simulink model "ResonantConverter_GaN"  (R2016a)
settings: Solver=VariableStepAuto  StartTime=0.0  StopTime=0.1  FixedStep=1e-6  RelTol=1e-3
libraries: powerlib x142, dspstat3 x22, powerlib_meascontrol x13
(part 2 of 2)

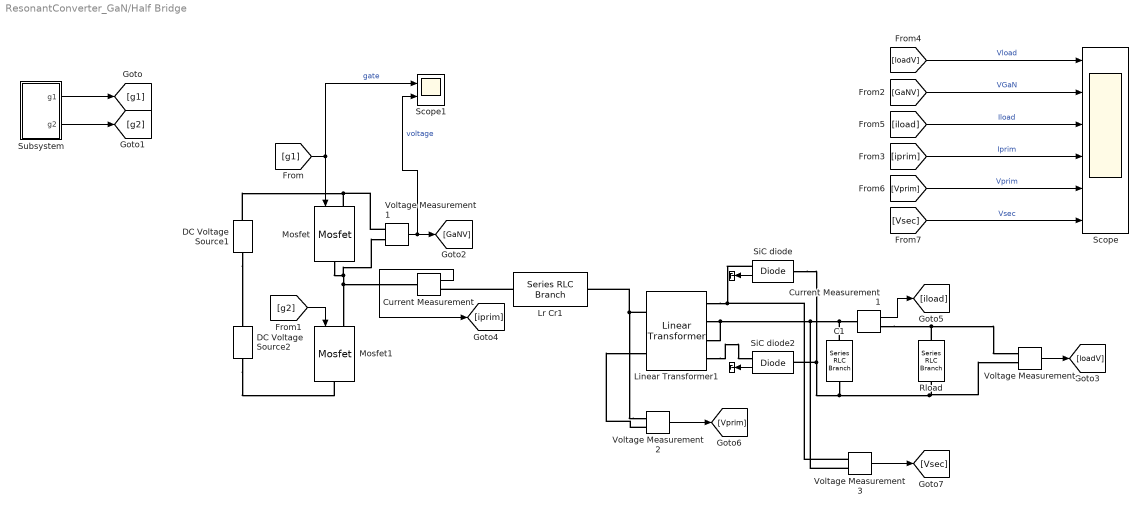
== system ResonantConverter_GaN/Half Bridge ==
  "  " : Terminator
  "   " : Terminator
  C1 : powerlib/Elements/Series RLC Branch  LConnTagsString=__new0  RConnTagsString=__new0  BranchType=C  Resistance=1  Inductance=1e-3  SetiL0=off  InitialCurrent=0  Capacitance=1e-6  Setx0=off  InitialVoltage=0  Measurements=None
  Current Measurement : powerlib/Measurements/Current Measurement  PhasorSimulation=off  OutputType=Complex  PSBequivalent=0
  Current Measurement1 : powerlib/Measurements/Current Measurement  PhasorSimulation=off  OutputType=Complex  PSBequivalent=0
  DC Voltage Source1 : powerlib/Electrical Sources/DC Voltage Source  Amplitude=190  Measurements=None
  DC Voltage Source2 : powerlib/Electrical Sources/DC Voltage Source  Amplitude=190  Measurements=None
  Linear Transformer1 : powerlib/Elements/Linear Transformer  UNITS=SI  NominalPower=[ 400 250e3 ]  winding1=[380 0.1805 4.5964e-06]  winding2=[380 0.1805 4.5964e-06]  ThreeWindings=on  winding3=[380 0.1805 4.5964e-06]  RmLm=[4e6 118e-06]  Measurements=None  DataType=on
  Lr Cr1 : powerlib/Elements/Series RLC Branch  LConnTagsString=__new0  RConnTagsString=__new0  BranchType=LC  Resistance=1  Inductance=100e-6  SetiL0=off  InitialCurrent=0  Capacitance=4.053e-10  Setx0=off  InitialVoltage=0  Measurements=None
  Mosfet : powerlib/Power Electronics/Mosfet  Ron=130e-3  Lon=0  Rd=0.25  Vfd=2.2  IC=0  Rs=1e5  Cs=inf  Measurements=off
  Mosfet1 : powerlib/Power Electronics/Mosfet  Ron=130e-3  Lon=0  Rd=0.25  Vfd=2.2  IC=0  Rs=1e5  Cs=inf  Measurements=off
  Rload : powerlib/Elements/Series RLC Branch  LConnTagsString=__new0  RConnTagsString=__new0  BranchType=R  Resistance=6  Inductance=1e-3  SetiL0=off  InitialCurrent=0  Capacitance=1e-6  Setx0=off  InitialVoltage=0  Measurements=None
  Scope : Scope  NumInputPorts=6
  Scope1 : Scope  NumInputPorts=2
  SiC diode : powerlib/Power Electronics/Diode  Ron=0.001  Lon=0  Vf=0.8  IC=0  UseSnubber=off  Rs=500  Cs=250e-9  Measurements=on
  SiC diode2 : powerlib/Power Electronics/Diode  Ron=0.001  Lon=0  Vf=0.8  IC=0  UseSnubber=off  Rs=500  Cs=250e-9  Measurements=on
  Subsystem : Subsystem
  Voltage Measurement{,1..3} (4 alike) : powerlib/Measurements/Voltage Measurement  PhasorSimulation=off  OutputType=Complex  PSBequivalent=0
  wires:
  Voltage Measurement/1 -> [loadV]
  [loadV] -> Scope/1  "Vload"
  [g2] -> Mosfet1/1
  [iprim] -> Scope/4  "Iprim"
  [g1] -> Mosfet/1, Scope1/1  "gate"
  Current Measurement1/1 -> [iload]
  [GaNV] -> Scope/2  "VGaN"
  Current Measurement/1 -> [iprim]
  SiC diode/1 -> "  "/1
  SiC diode2/1 -> "   "/1
  [iload] -> Scope/3  "Iload"
  Voltage Measurement1/1 -> [GaNV], Scope1/2  "voltage"
  Subsystem/1("g1 ") -> [g1]
  Subsystem/2(g2) -> [g2]
  Voltage Measurement2/1 -> [Vprim]
  [Vprim] -> Scope/5  "Vprim"
  Voltage Measurement3/1 -> [Vsec]
  [Vsec] -> Scope/6  "Vsec"
  connections:
  Linear Transformer1/RConn4 -- SiC diode2/RConn1
  Voltage Measurement2/LConn1 -- Linear Transformer1/LConn1 -- Lr Cr1/RConn1
  SiC diode/RConn1 -- Linear Transformer1/RConn1 -- Voltage Measurement3/LConn1
  SiC diode/LConn1 -- SiC diode2/LConn1 -- C1/RConn1 -- Voltage Measurement/LConn2 -- Rload/RConn1
  Voltage Measurement1/LConn1 -- DC Voltage Source1/RConn1 -- Mosfet/LConn1
  Rload/LConn1 -- Current Measurement1/RConn1 -- Voltage Measurement/LConn1
  Mosfet/RConn1 -- Mosfet1/LConn1 -- Current Measurement/LConn1 -- Voltage Measurement1/LConn2
  Linear Transformer1/RConn3 -- Linear Transformer1/RConn2 -- Voltage Measurement3/LConn2 -- C1/LConn1 -- Current Measurement1/LConn1
  Voltage Measurement2/LConn2 -- Linear Transformer1/LConn2
  Lr Cr1/LConn1 -- Current Measurement/RConn1
  DC Voltage Source1/LConn1 -- DC Voltage Source2/RConn1
  DC Voltage Source2/LConn1 -- Mosfet1/RConn1

== system ResonantConverter_GaN/230 khz Switch1/Subsystem ==
  Constant : Constant
  Constant1 : Constant  Value=0
  Constant2 : Constant  Value=0
  Constant3 : Constant
  Sawtooth Generator : powerlib_meascontrol/Pulse & Signal Generators/Sawtooth Generator  Freq=230e3  Phase=180  Ts=0
  Scope : Scope
  Switch : Switch  Criteria=u2 > Threshold
  Switch1 : Switch
  "g1 " : Outport
  g2 : Outport  Port=2
  wires:
  Constant/1 -> Switch/1
  Constant3/1 -> Switch1/3
  Constant1/1 -> Switch/3
  Constant2/1 -> Switch1/1
  Switch/1 -> "g1 "/1, Scope/1
  Sawtooth Generator/1 -> Switch/2, Switch1/2
  Switch1/1 -> g2/1

== system ResonantConverter_GaN/235 khz Switch3/Subsystem ==
  Constant : Constant
  Constant1 : Constant  Value=0
  Constant2 : Constant  Value=0
  Constant3 : Constant
  Sawtooth Generator : powerlib_meascontrol/Pulse & Signal Generators/Sawtooth Generator  Freq=235e3  Phase=180  Ts=0
  Scope : Scope
  Switch : Switch  Criteria=u2 > Threshold
  Switch1 : Switch
  "g1 " : Outport
  g2 : Outport  Port=2
  wires:
  Constant/1 -> Switch/1
  Constant3/1 -> Switch1/3
  Constant1/1 -> Switch/3
  Constant2/1 -> Switch1/1
  Switch/1 -> "g1 "/1, Scope/1
  Sawtooth Generator/1 -> Switch/2, Switch1/2
  Switch1/1 -> g2/1

== system ResonantConverter_GaN/238 khz Switch2/Subsystem ==
  Constant : Constant
  Constant1 : Constant  Value=0
  Constant2 : Constant  Value=0
  Constant3 : Constant
  Sawtooth Generator : powerlib_meascontrol/Pulse & Signal Generators/Sawtooth Generator  Freq=238e3  Phase=180  Ts=0
  Scope : Scope
  Switch : Switch  Criteria=u2 > Threshold
  Switch1 : Switch
  "g1 " : Outport
  g2 : Outport  Port=2
  wires:
  Switch1/1 -> g2/1
  Sawtooth Generator/1 -> Switch1/2, Switch/2
  Switch/1 -> Scope/1, "g1 "/1
  Constant2/1 -> Switch1/1
  Constant1/1 -> Switch/3
  Constant3/1 -> Switch1/3
  Constant/1 -> Switch/1

== system ResonantConverter_GaN/240 khz Switch2/Subsystem ==
  Constant : Constant
  Constant1 : Constant  Value=0
  Constant2 : Constant  Value=0
  Constant3 : Constant
  Sawtooth Generator : powerlib_meascontrol/Pulse & Signal Generators/Sawtooth Generator  Freq=240e3  Phase=180  Ts=0
  Scope : Scope
  Switch : Switch  Criteria=u2 > Threshold
  Switch1 : Switch
  "g1 " : Outport
  g2 : Outport  Port=2
  wires:
  Switch1/1 -> g2/1
  Sawtooth Generator/1 -> Switch1/2, Switch/2
  Switch/1 -> Scope/1, "g1 "/1
  Constant2/1 -> Switch1/1
  Constant1/1 -> Switch/3
  Constant3/1 -> Switch1/3
  Constant/1 -> Switch/1

== system ResonantConverter_GaN/241 khz Switch1/Subsystem ==
  Constant : Constant
  Constant1 : Constant  Value=0
  Constant2 : Constant  Value=0
  Constant3 : Constant
  Sawtooth Generator : powerlib_meascontrol/Pulse & Signal Generators/Sawtooth Generator  Freq=241e3  Phase=180  Ts=0
  Scope : Scope
  Switch : Switch  Criteria=u2 > Threshold
  Switch1 : Switch
  "g1 " : Outport
  g2 : Outport  Port=2
  wires:
  Switch1/1 -> g2/1
  Sawtooth Generator/1 -> Switch1/2, Switch/2
  Switch/1 -> Scope/1, "g1 "/1
  Constant2/1 -> Switch1/1
  Constant1/1 -> Switch/3
  Constant3/1 -> Switch1/3
  Constant/1 -> Switch/1

== system ResonantConverter_GaN/244 khz Switch1/Subsystem ==
  Constant : Constant
  Constant1 : Constant  Value=0
  Constant2 : Constant  Value=0
  Constant3 : Constant
  Sawtooth Generator : powerlib_meascontrol/Pulse & Signal Generators/Sawtooth Generator  Freq=244e3  Phase=180  Ts=0
  Scope : Scope
  Switch : Switch  Criteria=u2 > Threshold
  Switch1 : Switch
  "g1 " : Outport
  g2 : Outport  Port=2
  wires:
  Constant/1 -> Switch/1
  Constant3/1 -> Switch1/3
  Constant1/1 -> Switch/3
  Constant2/1 -> Switch1/1
  Switch/1 -> "g1 "/1, Scope/1
  Sawtooth Generator/1 -> Switch/2, Switch1/2
  Switch1/1 -> g2/1

== system ResonantConverter_GaN/245 khz Switch1/Subsystem ==
  Constant : Constant
  Constant1 : Constant  Value=0
  Constant2 : Constant  Value=0
  Constant3 : Constant
  Sawtooth Generator : powerlib_meascontrol/Pulse & Signal Generators/Sawtooth Generator  Freq=245e3  Phase=180  Ts=0
  Scope : Scope
  Switch : Switch  Criteria=u2 > Threshold
  Switch1 : Switch
  "g1 " : Outport
  g2 : Outport  Port=2
  wires:
  Constant/1 -> Switch/1
  Constant3/1 -> Switch1/3
  Constant1/1 -> Switch/3
  Constant2/1 -> Switch1/1
  Switch/1 -> "g1 "/1, Scope/1
  Sawtooth Generator/1 -> Switch/2, Switch1/2
  Switch1/1 -> g2/1

== system ResonantConverter_GaN/247 khz Switch2/Subsystem ==
  Constant : Constant
  Constant1 : Constant  Value=0
  Constant2 : Constant  Value=0
  Constant3 : Constant
  Sawtooth Generator : powerlib_meascontrol/Pulse & Signal Generators/Sawtooth Generator  Freq=247e3  Phase=180  Ts=0
  Scope : Scope
  Switch : Switch  Criteria=u2 > Threshold
  Switch1 : Switch
  "g1 " : Outport
  g2 : Outport  Port=2
  wires:
  Switch1/1 -> g2/1
  Sawtooth Generator/1 -> Switch1/2, Switch/2
  Switch/1 -> Scope/1, "g1 "/1
  Constant2/1 -> Switch1/1
  Constant1/1 -> Switch/3
  Constant3/1 -> Switch1/3
  Constant/1 -> Switch/1

== system ResonantConverter_GaN/250 khz Switch/Subsystem ==
  Constant : Constant
  Constant1 : Constant  Value=0
  Constant2 : Constant  Value=0
  Constant3 : Constant
  Sawtooth Generator : powerlib_meascontrol/Pulse & Signal Generators/Sawtooth Generator  Freq=250e3  Phase=180  Ts=0
  Scope : Scope
  Switch : Switch  Criteria=u2 > Threshold
  Switch1 : Switch
  "g1 " : Outport
  g2 : Outport  Port=2
  wires:
  Switch1/1 -> g2/1
  Sawtooth Generator/1 -> Switch1/2, Switch/2
  Switch/1 -> Scope/1, "g1 "/1
  Constant2/1 -> Switch1/1
  Constant1/1 -> Switch/3
  Constant3/1 -> Switch1/3
  Constant/1 -> Switch/1

== system ResonantConverter_GaN/250 khz Switch1/Subsystem ==
  Constant : Constant
  Constant1 : Constant  Value=0
  Constant2 : Constant  Value=0
  Constant3 : Constant
  Sawtooth Generator : powerlib_meascontrol/Pulse & Signal Generators/Sawtooth Generator  Freq=250e3  Phase=180  Ts=0
  Scope : Scope
  Switch : Switch  Criteria=u2 > Threshold
  Switch1 : Switch
  "g1 " : Outport
  g2 : Outport  Port=2
  wires:
  Constant/1 -> Switch/1
  Constant3/1 -> Switch1/3
  Constant1/1 -> Switch/3
  Constant2/1 -> Switch1/1
  Switch/1 -> "g1 "/1, Scope/1
  Sawtooth Generator/1 -> Switch/2, Switch1/2
  Switch1/1 -> g2/1

== system ResonantConverter_GaN/250 khz Switch2/Subsystem ==
  Constant : Constant
  Constant1 : Constant  Value=0
  Constant2 : Constant  Value=0
  Constant3 : Constant
  Sawtooth Generator : powerlib_meascontrol/Pulse & Signal Generators/Sawtooth Generator  Freq=250e3  Phase=180  Ts=0
  Scope : Scope
  Switch : Switch  Criteria=u2 > Threshold
  Switch1 : Switch
  "g1 " : Outport
  g2 : Outport  Port=2
  wires:
  Switch1/1 -> g2/1
  Sawtooth Generator/1 -> Switch1/2, Switch/2
  Switch/1 -> Scope/1, "g1 "/1
  Constant2/1 -> Switch1/1
  Constant1/1 -> Switch/3
  Constant3/1 -> Switch1/3
  Constant/1 -> Switch/1

== system ResonantConverter_GaN/Half Bridge/Subsystem ==
  Constant : Constant
  Constant1 : Constant  Value=0
  Constant2 : Constant  Value=0
  Constant3 : Constant
  On Delay : powerlib_meascontrol/Logic/On Delay  DelayType=On delay  delay=0.5e-5/(250e3)  ic=0  Ts=0
  Sawtooth Generator : powerlib_meascontrol/Pulse & Signal Generators/Sawtooth Generator  Freq=250e3  Phase=180  Ts=0
  Switch : Switch  Criteria=u2 > Threshold
  Switch1 : Switch
  "g1 " : Outport
  g2 : Outport  Port=2
  wires:
  Sawtooth Generator/1 -> Switch1/2, Switch/2
  Switch/1 -> "g1 "/1
  Constant2/1 -> Switch1/1
  Constant1/1 -> Switch/3
  Constant3/1 -> Switch1/3
  Constant/1 -> Switch/1
  Switch1/1 -> On Delay/1
  On Delay/1 -> g2/1
